simulink model "Bai2_TricycleBabyDrive"  (R2018a)
settings: Solver=ode15s  StartTime=0.0  StopTime=1000  RelTol=1e-3
libraries: simulink x1
settings Model: Creator=Administrator  LastModifiedBy=Administrator
settings SolverCC: AlgebraicLoopSolver=LineSearch
settings DebuggingCC: ParameterPrecisionLossMsg=none

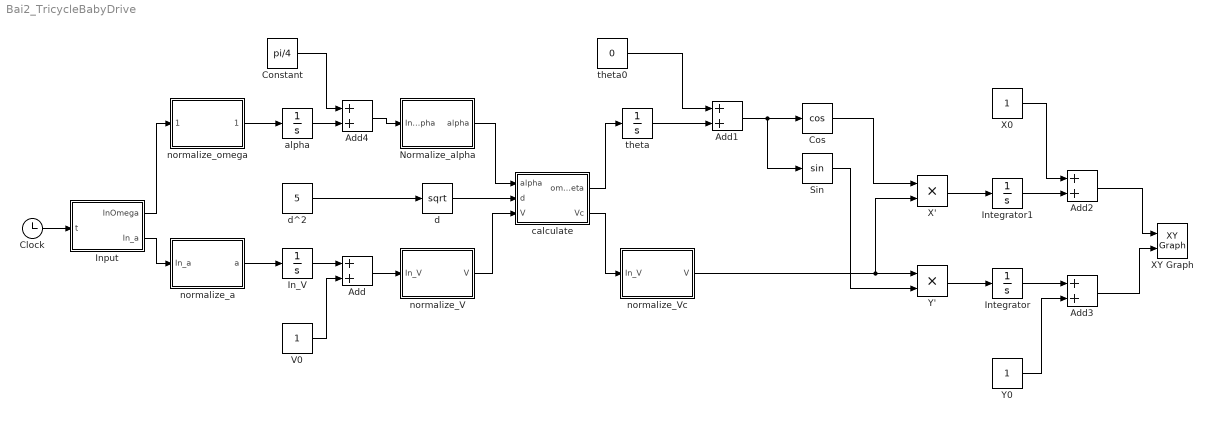
== system Bai2_TricycleBabyDrive ==
  Add{,1..4} (5 alike) : Sum
  Clock : Clock
  Constant : Constant  Value=pi/4
  Cos : Trigonometry  Operator=cos
  In_V : Integrator
  Input : MATLAB Function  TreatAsAtomicUnit=on
  Integrator : Integrator
  Integrator1 : Integrator
  Normalize_alpha : MATLAB Function  TreatAsAtomicUnit=on
  Sin : Trigonometry
  V0 : Constant
  X' : Product
  X0 : Constant
  XY Graph : simulink/Sinks/XY Graph  xmin=-10  xmax=10  ymin=-10  ymax=10  st=-1
  Y' : Product
  Y0 : Constant
  alpha : Integrator
  calculate : MATLAB Function  TreatAsAtomicUnit=on
  d : Sqrt  SaturateOnIntegerOverflow=on
  "d^2 " : Constant  Value=5
  normalize_V : MATLAB Function  TreatAsAtomicUnit=on
  normalize_Vc : MATLAB Function  TreatAsAtomicUnit=on
  normalize_a : MATLAB Function  TreatAsAtomicUnit=on
  normalize_omega : MATLAB Function  TreatAsAtomicUnit=on
  theta : Integrator
  theta0 : Constant  Value=0
  wires:
  Clock/1 -> Input/1(t)
  Input/2(In_a) -> normalize_a/1(In_a)
  normalize_a/1(a) -> In_V/1
  In_V/1 -> Add/1
  Add/1 -> normalize_V/1(In_V)
  V0/1 -> Add/2
  theta0/1 -> Add1/1
  Add1/1 -> Sin/1, Cos/1
  Sin/1 -> Y'/2
  Cos/1 -> X'/1
  "d^2 "/1 -> d/1
  Y'/1 -> Integrator/1
  X'/1 -> Integrator1/1
  Integrator1/1 -> Add2/2
  Integrator/1 -> Add3/1
  Y0/1 -> Add3/2
  X0/1 -> Add2/1
  Add2/1 -> XY Graph/1
  Add3/1 -> XY Graph/2
  normalize_Vc/1(V) -> Y'/1, X'/2
  Input/1(InOmega) -> normalize_omega/1(InOmega)
  normalize_omega/1(Omega) -> alpha/1
  Normalize_alpha/1(alpha) -> calculate/1(alpha)
  d/1 -> calculate/2(d)
  normalize_V/1(V) -> calculate/3(V)
  calculate/1(omega_theta) -> theta/1
  theta/1 -> Add1/2
  calculate/2(Vc) -> normalize_Vc/1(In_V)
  alpha/1 -> Add4/2
  Add4/1 -> Normalize_alpha/1(In_alpha)
  Constant/1 -> Add4/1

== matlab function Bai2_TricycleBabyDrive/normalize_omega ==
  data: InOmega input; Omega output
function Omega = fcn(InOmega)

if(InOmega >= 0.3) Omega = 0.3;
elseif(InOmega <= -0.3) Omega = -0.3;
else Omega = InOmega;
end

== matlab function Bai2_TricycleBabyDrive/Input ==
  data: t input; InOmega output; In_a output
function [InOmega, In_a]= fcn(t)

% a) Van toc va goc lai co dinh
InOmega = 0;
In_a = 0;

% b) Van toc co dinh va goc lai thay doi theo thoi gian
%InOmega = 0.05;
%In_a = 0;

% c) Van toc và goc lai thay doi theo thoi gian
%InOmega = 0.05;
%In_a = 0.1;

== matlab function Bai2_TricycleBabyDrive/normalize_a ==
  data: In_a input; a output
function a = fcn(In_a)

if(In_a >= 0.45) a = 0.45;
elseif(In_a <= -0.45) a = -0.45;
else a = In_a;
end

== matlab function Bai2_TricycleBabyDrive/normalize_V ==
  data: In_V input; V output
function V = fcn(In_V)

if(In_V >= 2.25) V = 2.25;
elseif(In_V <=-2.25) V = -2.25;
else V = In_V;
end

== matlab function Bai2_TricycleBabyDrive/Normalize_alpha ==
  data: In_alpha input; alpha output
function alpha = fcn(In_alpha)

if(In_alpha >= 3.14/4) alpha = 3.14/4;
elseif(In_alpha <= -3.14/4) alpha = -3.14/4;
else alpha = In_alpha;
end

== matlab function Bai2_TricycleBabyDrive/normalize_Vc ==
  data: In_V input; V output
function V = fcn(In_V)

if(In_V >= 2.25) V = 2.25;
elseif(In_V <=-2.25) V = -2.25;
else V = In_V;
end

== matlab function Bai2_TricycleBabyDrive/calculate ==
  data: alpha input; d input; omega_theta output; V input; Vc output
function [omega_theta, Vc] = fcn(alpha, d, V)

if(alpha == 0)
    omega_theta = 0;
    Vc = V;
else
    R = d/tan(alpha);
    omega_theta = V / sqrt(d^2 + R^2);
    Vc = omega_theta * R;
end
